simulink model "final_glimberg_104410"  (R2021a)
settings: Solver=VariableStepAuto  StartTime=0.0  StopTime=10.0  RelTol=1e-3
settings Model: Creator=pedro  LastModifiedBy=user

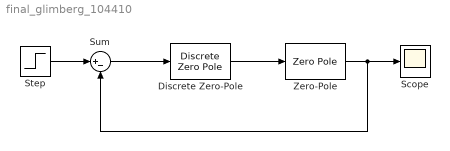
== system final_glimberg_104410 ==
  Discrete Zero-Pole : DiscreteZeroPole  Zeros=[-4]  Poles=[0]  Gain=40  SampleTime=-1
  Scope : Scope
  Step : Step  After=2*pi/180  SampleTime=0
  Sum : Sum  Inputs=|+-
  Zero-Pole : ZeroPole  Zeros=[-2 -2]  Poles=[0 4 4]  ContinuousStateAttributes='Planta'
  wires:
  Step/1 -> Sum/1
  Sum/1 -> Discrete Zero-Pole/1
  Discrete Zero-Pole/1 -> Zero-Pole/1
  Zero-Pole/1 -> Sum/2, Scope/1
